simulink library "lowLevel"  (R2017a)
settings: Solver=VariableStepAuto  StartTime=0.0  StopTime=10.0  RelTol=1e-3
settings Model: Creator=M.Cobb  LastModifiedBy=mitchell

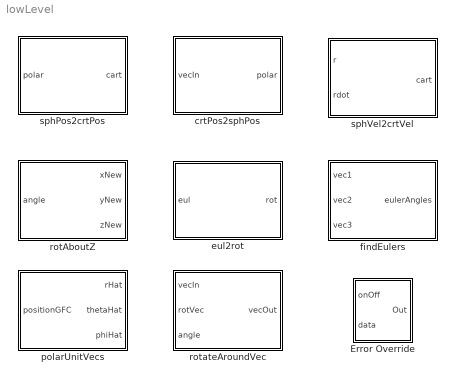
== system lowLevel ==
  Error Override : Subsystem
  crtPos2sphPos : MATLAB Function  TreatAsAtomicUnit=on
  eul2rot : MATLAB Function  TreatAsAtomicUnit=on
  findEulers : MATLAB Function  TreatAsAtomicUnit=on
  polarUnitVecs : MATLAB Function  TreatAsAtomicUnit=on
  rotAboutZ : MATLAB Function  TreatAsAtomicUnit=on
  rotateAroundVec : MATLAB Function  TreatAsAtomicUnit=on
  sphPos2crtPos : MATLAB Function  TreatAsAtomicUnit=on
  sphVel2crtVel : MATLAB Function  TreatAsAtomicUnit=on

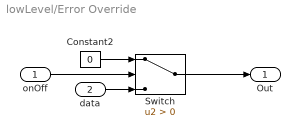
== system lowLevel/Error Override ==
  onOff : Inport
  data : Inport  Port=2
  Constant2 : Constant  Value=0
  Switch : Switch  Criteria=u2 > Threshold
  Out : Outport
  wires:
  Switch/1 -> Out/1
  onOff/1 -> Switch/2
  Constant2/1 -> Switch/1
  data/1 -> Switch/3

== matlab function lowLevel/sphVel2crtVel ==
  data: r input; cart output; rdot input
function cart = sphVel2crtVel(r,rdot)
% convert a ground fixed polar vector to ground fixed cartesian
% This follows the wolfram convention outlined here:
% http://mathworld.wolfram.com/SphericalCoordinates.html
cart = [0;0;0];
cart(1) =       cos(r(2))*sin(r(3))*rdot(1)...
          -r(1)*sin(r(2))*sin(r(3))*rdot(2)...
          +r(1)*cos(r(2))*cos(r(3))*rdot(3);

cart(2) =       sin(r(2))*sin(r(3))*rdot(1)...
          +r(1)*cos(r(2))*sin(r(3))*rdot(2)...
          +r(1)*sin(r(2))*cos(r(3))*rdot(3);

cart(3) = cos(r(3))*rdot(1)-r(1)*sin(r(3))*rdot(3);
end

== matlab function lowLevel/eul2rot ==
  data: eul input; rot output
function rot = eul2rot(eul)
% Convert Euler angles to rotation Matrix
% yaw   = [cos(eul(1)) -sin(eul(1)) 0; sin(eul(1)) cos(eul(1)) 0;0 0 1];
% pitch = [cos(eul(2)) 0 sin(eul(2));0 1 0; -sin(eul(2)) 0 cos(eul(2))];
% roll  = [1 0 0;0 cos(eul(3)) -sin(eul(3));0 sin(eul(3)) cos(eul(3))];
% rot = roll*pitch*yaw;
rot = eul2rotm(eul','ZYX');
end

== matlab function lowLevel/crtPos2sphPos ==
  data: vecIn input; polar output
function polar = cart2sphere(vecIn)
% convert a cartesian vector to a spherical vector
% this follows the conventioned outlined here: 
% http://mathworld.wolfram.com/SphericalCoordinates.html
polar = [0;0;0];
% polar(1) = sqrt(sum(cart.^2));
% polar(2) = atan2(cart(2),cart(1));
% polar(3) = (pi/2)-acos(cart(3)/polar(1));
polar(1) = sqrt(sum(vecIn.^2));         %r
polar(2) = atan2(vecIn(2),vecIn(1));    %theta
polar(3) = acos(vecIn(3)/polar(1));            %phi
end

== matlab function lowLevel/sphPos2crtPos ==
  data: polar input; cart output
function cart = sphere2cart(polar)
% convert a ground fixed polar vector to ground fixed cartesian
% This follows the wolfram convention outlined here:
% http://mathworld.wolfram.com/SphericalCoordinates.html
cart = [0;0;0];
cart(1) = polar(1)*cos(polar(2))*sin(polar(3));
cart(2) = polar(1)*sin(polar(2))*sin(polar(3));
cart(3) = polar(1)*cos(polar(3));
end

== matlab function lowLevel/polarUnitVecs ==
  data: positionGFC input; rHat output; thetaHat output; phiHat output
function [rHat,thetaHat,phiHat] = polarUnitVecs(positionGFC)
% Find ground-frame representation of spherical unit vectors for a given
% cartesian vector.  Each unit vector output is represented in ground frame
% cartesian components This follows the wolfram convention outlined here:
% http://mathworld.wolfram.com/SphericalCoordinates.html
r       = sqrt(sum(positionGFC.^2));
theta   = atan2(positionGFC(2),positionGFC(1));
phi     = acos(positionGFC(3)/r);

rHat        = [cos(theta)*sin(phi)  sin(theta)*sin(phi) cos(phi)    ]';
thetaHat    = [-sin(theta)          cos(theta)          0           ]';
phiHat      = [cos(theta)*cos(phi)  sin(theta)*cos(phi) -sin(phi)   ]';
end

== matlab function lowLevel/rotAboutZ ==
  data: angle input; xNew output; yNew output; zNew output
function [xNew,yNew,zNew] = rotAboutZ(angle)
% Function takes the body fixed x, y, anz axes and rotates them about the z
% axis by the amount specified in angle.
xHat = [1 0 0]';
yHat = [0 1 0]';
zHat = [0 0 1]';
R = [cos(angle),-sin(angle) 0;sin(angle) cos(angle) 0;0 0 1];
xNew = R*xHat;
yNew = R*yHat;
zNew = R*zHat;

end

== matlab function lowLevel/findEulers ==
  data: vec1 input; eulerAngles output; vec2 input; vec3 input
function eulerAngles = findEulers(vec1,vec2,vec3)
% Function takes the sperical thetaHat and phiHat and rotates about the
% rHat vector by the amount specified in angle.  Returns 3 3-element column
% vectors representing the new vectors in spherical coordinates.
rHat = [1 0 0]';
thetaHat = [0 1 0]';
phiHat = [0 0 1]';
rot = [cos(angle) -sin(angle) 0; sin(angle) cos(angle) 0;0 0 1];
rNew = rot*rHat;
thetaNew = rot*thetaHat;
phiNew = rot*phiHat;
end

== matlab function lowLevel/rotateAroundVec ==
  data: vecIn input; vecOut output; rotVec input; angle input
function vecOut = rotateAroundVec(vecIn,rotVec,angle)
% Function rotates a vector around an arbitrary vector.
% vecIn = vector to be rotated
% rotVec = vector that defines the axis of rotation
% angle = the angle of rotation
% vecOut = angle after rotation
% This follows the procedure outlined here:
% http://ksuweb.kennesaw.edu/~plaval//math4490/rotgen.pdf
% position=vecIn';
% T=[1 0 0 -position(1);0 1 0 -position(2);0 0 1 -position(3);0 0 0 1];
% Tinv=[1 0 0 position(1);0 1 0 position(2);0 0 1 position(3);0 0 0 1];
% vecIn = [vecIn(1) vecIn(2) vecIn(3) 1]./sqrt(sum(vecIn.^2));
% vecOut = zeros(3,1);
% a = rotVec(1);
% b = rotVec(2);
% c = rotVec(3);
% d = sqrt(b^2+c^2);
% if d~=0
%     Rx = [1 0 0 0;0 c/d -b/d 0;0 b/d c/d 0;0 0 0 1];
%     RxInv = Rx';
%     Ry = [d 0 -a 0;0 1 0 0;a 0 d 0;0 0 0 1];
%     RyInv = Ry';
%     Rz=[cos(angle) -sin(angle) 0 0;sin(angle) cos(angle) 0 0;0 0 1 0;0 0 0 1];
%     vec = Tinv*RxInv*RyInv*Rz*Ry*Rx*T*vecIn';
%     vecOut = [vec(1) vec(2) vec(3)]';
% else
%     vecOut = position';
% end

C=cos(angle);
S=sin(angle);
t=1-cos(angle);
r=rotVec./sqrt(sum(rotVec.^2));
ux=r(1);uy=r(2);uz=r(3);
R=[t*ux^2+C        t*ux*uy-S*uz    t*ux*uz+S*uy;...
   t*ux*uy+S*uz    t*uy^2+C        t*uy*uz-S*ux;...
   t*ux*uz-S*uy    t*uy*uz+S*ux    t*uz^2+C];
vecOutTranspose = R*[vecIn(1);vecIn(2);vecIn(3)];
vecOut = vecOutTranspose';
end
